simulink model "db_pend_cart_lin"  (R2020a)
settings: Solver=VariableStepAuto  StartTime=0.0  StopTime=60  RelTol=1e-3
values from neighbouring files (symbols this model uses):
  g = 9.81    [cannonballpar.m]    (also in pendcartpar.m = 1; pendragpar.m)
  l = 1    [pend4par.m]    (also in pendcartpar.m; pendragpar.m = 0.1)
  m = 1    [cannonballpar.m]    (also in pendcartpar.m; pendragpar.m = 0.01)
undefined symbols (not defined in the file or in its folder): theta1e, theta2e, ye
settings Model: Creator=Tomo  LastModifiedBy=Tomo
settings OptimizationCC: DefaultParameterBehavior=Inlined  BufferReuse=off
settings DebuggingCC: InitInArrayFormatMsg=none

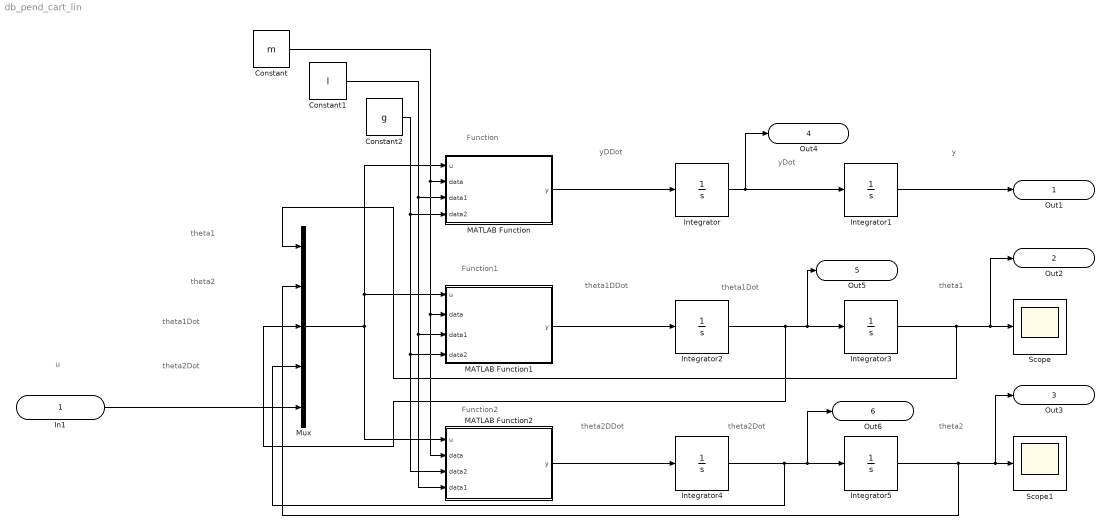
== system db_pend_cart_lin ==
  note: Function
  note: y
  note: yDot
  note: yDDot
  note: theta1
  note: theta2
  note: theta1Dot
  note: theta1DDot
  note: theta2DDot
  note: theta2Dot
  note: theta1
  note: theta2
  note: theta1Dot
  note: theta2Dot
  note: u
  note: Function1
  note: Function2
  In1 : Inport
  Constant : Constant  Value=m  VectorParams1D=off
  Constant1 : Constant  Value=l  VectorParams1D=off
  Constant2 : Constant  Value=g  VectorParams1D=off
  Integrator : Integrator
  Integrator1 : Integrator  InitialCondition=ye
  Integrator2 : Integrator
  Integrator3 : Integrator  InitialCondition=theta1e
  Integrator4 : Integrator
  Integrator5 : Integrator  InitialCondition=theta2e
  MATLAB Function : MATLAB Function  TreatAsAtomicUnit=on
  MATLAB Function1 : MATLAB Function  TreatAsAtomicUnit=on
  MATLAB Function2 : MATLAB Function  TreatAsAtomicUnit=on
  Mux : Mux  Inputs=5
  Scope : Scope
  Scope1 : Scope
  Out1 : Outport
  Out2 : Outport  Port=2
  Out3 : Outport  Port=3
  Out4 : Outport  Port=4
  Out5 : Outport  Port=5
  Out6 : Outport  Port=6
  wires:
  In1/1 -> Mux/5
  MATLAB Function1/1(y) -> Integrator2/1
  Integrator2/1 -> Mux/3, Out5/1, Integrator3/1
  Integrator3/1 -> Mux/1, Out2/1, Scope/1
  MATLAB Function2/1(y) -> Integrator4/1
  Integrator5/1 -> Mux/2, Out3/1, Scope1/1
  MATLAB Function/1(y) -> Integrator/1
  Integrator/1 -> Out4/1, Integrator1/1
  Integrator1/1 -> Out1/1
  Constant/1 -> MATLAB Function2/2(data), MATLAB Function1/2(data), MATLAB Function/2(data)
  Constant1/1 -> MATLAB Function2/4(data1), MATLAB Function1/3(data1), MATLAB Function/3(data1)
  Constant2/1 -> MATLAB Function2/3(data2), MATLAB Function1/4(data2), MATLAB Function/4(data2)
  Mux/1 -> MATLAB Function/1(u), MATLAB Function1/1(u), MATLAB Function2/1(u)
  Integrator4/1 -> Mux/4, Out6/1, Integrator5/1

== matlab function db_pend_cart_lin/MATLAB Function1 ==
  data: u input size=5; y output; data input; data1 input; data2 input
function y = fcn(u, data, data1, data2)
    %{
        EMBEDDED MATLAB BLOCK FUNCTION1
    %}
    m0 = data(1); m1 = data(2); m2 = data(3); l1 = data1(1); l2 = data1(2);
    g = data2;
    
    num = -(m1*l1*cos(u(1))*sin(u(1))*u(3)*u(3) + m2*l2*cos(u(1))*sin(u(2))*u(4)*u(4))...
            + m2*g*(sin(u(1))*cos(u(2))^2 - cos(u(1))*sin(u(2))*cos(u(2)))...
            - (m0 + m1 + m2)*g*sin(u(1)) + u(5)*cos(u(1));
    den = l1*(m0 + m1 + m2 - m1*cos(u(1))^2 - m2*cos(u(2))^2);
    y = num / den;
end

== matlab function db_pend_cart_lin/MATLAB Function ==
  data: u input size=5; y output; data input; data1 input; data2 input
function y = fcn(u, data, data1, data2)
    %{
        EMBEDDED MATLAB BLOCK FUNCTION
    %}
    
    m0 = data(1); m1 = data(2); m2 = data(3); l1 = data1(1); l2 = data1(2);
    g = data2;
    
    num = -m1*l1*sin(u(1))*u(3)*u(3) - m2*l2*sin(u(2))*u(4)*u(4)...
            - m1*g*sin(u(1))*cos(u(1)) - m2*g*sin(u(2))*cos(u(2))...
            + u(5);
    den = m0 + m1 + m2 - m1*cos(u(1))^2 - m2*cos(u(2))^2;
    y = num / den;
end

== matlab function db_pend_cart_lin/MATLAB Function2 ==
  data: u input size=5; y output; data input; data2 input; data1 input
function y = fcn(u, data, data2, data1)
    %{
        EMBEDDED MATLAB BLOCK FUNCTION2
    %}
    m0 = data(1); m1 = data(2); m2 = data(3); l1 = data1(1); l2 = data1(2);
    g = data2;
    
    num = -(m1*l1*cos(u(2,1))*sin(u(1))*u(3)*u(3) + m2*l2*cos(u(2))*sin(u(2))*u(4)*u(4))...
            + m1*g*(sin(u(2))*cos(u(1))^2 - cos(u(2))*sin(u(1))*cos(u(1)))...
            - (m0 + m1 + m2)*g*sin(u(2)) + u(5)*cos(u(2));
    den = l2*(m0 + m1 + m2 - m1*cos(u(1))^2 - m2*cos(u(2))^2);
    y = num / den;
end
